simulink model "s12_euler_ssprk3_muscl_minmod_pp_ref"  (R2026a)
settings: Solver=FixedStepDiscrete  StopTime=0  FixedStep=1
model workspace (MAT data in the model file):
  S12_PP_CFLHardMax = 0.5
  S12_PP_PFloor = 1e-13
  S12_PP_RhoFloor = 1e-13
  S12_RK3_CFL = Simulink.Parameter
  S12_RK3_CFL.Value = 0.45
  S12_RK3_CFL.Complexity = 'real'
  S12_RK3_CFL.Dimensions = [1 1]
  S12_RK3_CFL.Description = 'CFL stability factor.'
  S12_RK3_CFL.DataType = 'auto'
  S12_RK3_Dx = Simulink.Parameter
  S12_RK3_Dx.Value = 0.005
  S12_RK3_Dx.Complexity = 'real'
  S12_RK3_Dx.Dimensions = [1 1]
  S12_RK3_Dx.Description = 'Uniform cell width.'
  S12_RK3_Dx.DataType = 'auto'
  S12_RK3_EndTime = Simulink.Parameter
  S12_RK3_EndTime.Value = 0.2
  S12_RK3_EndTime.Complexity = 'real'
  S12_RK3_EndTime.Dimensions = [1 1]
  S12_RK3_EndTime.Description = 'Integration end time.'
  S12_RK3_EndTime.DataType = 'auto'
  S12_RK3_Gamma = Simulink.Parameter
  S12_RK3_Gamma.Value = 1.4
  S12_RK3_Gamma.Complexity = 'real'
  S12_RK3_Gamma.Dimensions = [1 1]
  S12_RK3_Gamma.Description = 'Ratio of specific heats.'
  S12_RK3_Gamma.DataType = 'auto'
  S12_RK3_MaxSteps = Simulink.Parameter
  S12_RK3_MaxSteps.Value = 10000
  S12_RK3_MaxSteps.Complexity = 'real'
  S12_RK3_MaxSteps.Dimensions = [1 1]
  S12_RK3_MaxSteps.Description = 'Maximum accepted SSP-RK3 steps.'
  S12_RK3_MaxSteps.DataType = 'auto'
  S12_RK3_State = Simulink.Parameter
  S12_RK3_State.Value = [1 0 2.5 1 0 2.5 1 0 2.5 1 0 2.5 ... (600 elements, 3x200)]
  S12_RK3_State.Complexity = 'real'
  S12_RK3_State.Dimensions = [3 200]
  S12_RK3_State.Description = 'Classic Sod conservative state [rho; rho*u; rho*E], 3x200.'
  S12_RK3_State.DataType = 'auto'
settings Model: Creator=Jovi  LastModifiedBy=Jovi

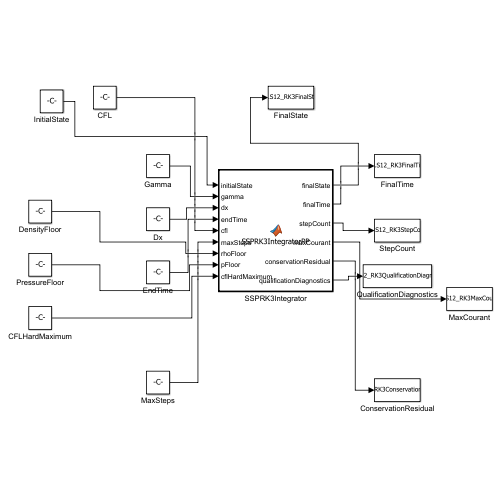
[thumbnail: Simulink's stored preview of the top-level diagram]
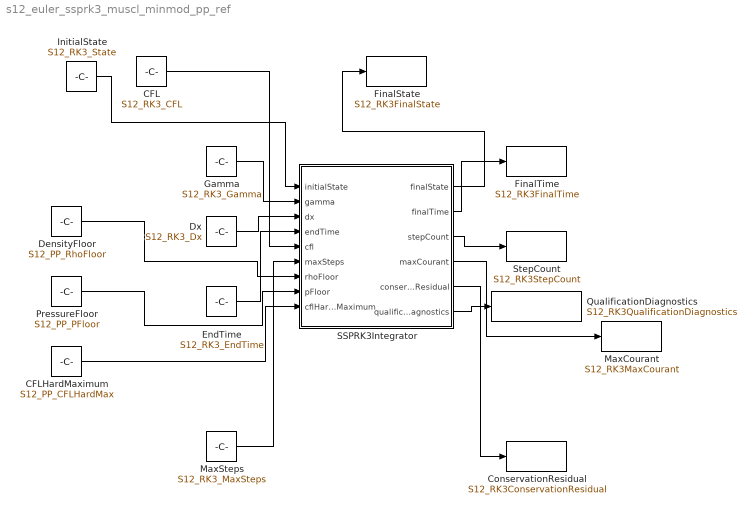
== system s12_euler_ssprk3_muscl_minmod_pp_ref ==
  CFL : Constant  Value=S12_RK3_CFL
  CFLHardMaximum : Constant  Value=S12_PP_CFLHardMax
  ConservationResidual : ToWorkspace  VariableName=S12_RK3ConservationResidual  SampleTime=-1
  DensityFloor : Constant  Value=S12_PP_RhoFloor
  Dx : Constant  Value=S12_RK3_Dx
  EndTime : Constant  Value=S12_RK3_EndTime
  FinalState : ToWorkspace  VariableName=S12_RK3FinalState  SampleTime=-1
  FinalTime : ToWorkspace  VariableName=S12_RK3FinalTime  SampleTime=-1
  Gamma : Constant  Value=S12_RK3_Gamma
  InitialState : Constant  Value=S12_RK3_State
  MaxCourant : ToWorkspace  VariableName=S12_RK3MaxCourant  SampleTime=-1
  MaxSteps : Constant  Value=S12_RK3_MaxSteps
  PressureFloor : Constant  Value=S12_PP_PFloor
  QualificationDiagnostics : ToWorkspace  VariableName=S12_RK3QualificationDiagnostics
  SSPRK3Integrator : MATLAB Function  TreatAsAtomicUnit=on
  StepCount : ToWorkspace  VariableName=S12_RK3StepCount  SampleTime=-1
  wires:
  InitialState/1 -> SSPRK3Integrator/1(initialState)
  Gamma/1 -> SSPRK3Integrator/2(gamma)
  Dx/1 -> SSPRK3Integrator/3(dx)
  EndTime/1 -> SSPRK3Integrator/4(endTime)
  CFL/1 -> SSPRK3Integrator/5(cfl)
  MaxSteps/1 -> SSPRK3Integrator/6(maxSteps)
  SSPRK3Integrator/1(finalState) -> FinalState/1
  SSPRK3Integrator/2(finalTime) -> FinalTime/1
  SSPRK3Integrator/3(stepCount) -> StepCount/1
  SSPRK3Integrator/4(maxCourant) -> MaxCourant/1
  SSPRK3Integrator/5(conservationResidual) -> ConservationResidual/1
  SSPRK3Integrator/6(qualificationDiagnostics) -> QualificationDiagnostics/1
  DensityFloor/1 -> SSPRK3Integrator/7(rhoFloor)
  PressureFloor/1 -> SSPRK3Integrator/8(pFloor)
  CFLHardMaximum/1 -> SSPRK3Integrator/9(cflHardMaximum)

== matlab function s12_euler_ssprk3_muscl_minmod_pp_ref/SSPRK3Integrator ==
  data: initialState input; finalState output; gamma input; dx input; endTime input; cfl input; maxSteps input; finalTime output; stepCount output; maxCourant output; conservationResidual output; qualificationDiagnostics output; rhoFloor input; pFloor input; cflHardMaximum input
function [finalState,finalTime,stepCount,maxCourant,conservationResidual,qualificationDiagnostics] = SSPRK3IntegratorPP(initialState,gamma,dx,endTime,cfl,maxSteps,rhoFloor,pFloor,cflHardMaximum)
%#codegen
cflTarget = 0.45;
maximumRetries = 8;
validateState(initialState,gamma,rhoFloor,pFloor);
U = initialState;
time = 0;
stepCount = 0;
maxCourant = 0;
boundaryIntegral = zeros(3,1);
qualificationDiagnostics = [inf,inf,0,0,0,0,0,0,0,0,0,1,0,0,0,1,inf,inf,inf,inf,0,0,0,0,0,inf(1,24)];
while time < endTime
    if stepCount >= maxSteps
        error('S12:Positivity:MaxSteps','PP SSP-RK3 exhausted maxSteps.');
    end
    alphaBase = stageAlpha(U,gamma);
    nominalDt = cfl*dx/alphaBase;
    dt = min(nominalDt,endTime-time);
    endClipped = dt < nominalDt;
    accepted = false;
    for attempt = 0:maximumRetries
        alpha0 = stageAlpha(U,gamma);
        if dt*alpha0/dx > cflHardMaximum
            qualificationDiagnostics(24) = qualificationDiagnostics(24)+1;
            qualificationDiagnostics(25) = qualificationDiagnostics(25)+1;
            dt = cflTarget*dx/alpha0;
            continue
        end
        [euler0,left0,right0,d0] = forwardEuler(U,gamma,dx,dt,rhoFloor,pFloor);
        U1 = euler0;
        validateState(U1,gamma,rhoFloor,pFloor);
        alpha1 = stageAlpha(U1,gamma);
        if dt*alpha1/dx > cflHardMaximum
            qualificationDiagnostics(24) = qualificationDiagnostics(24)+1;
            qualificationDiagnostics(25) = qualificationDiagnostics(25)+1;
            dt = cflTarget*dx/alpha1;
            continue
        end
        [euler1,left1,right1,d1] = forwardEuler(U1,gamma,dx,dt,rhoFloor,pFloor);
        U2 = 0.75*U+0.25*euler1;
        validateState(U2,gamma,rhoFloor,pFloor);
        alpha2 = stageAlpha(U2,gamma);
        if dt*alpha2/dx > cflHardMaximum
            qualificationDiagnostics(24) = qualificationDiagnostics(24)+1;
            qualificationDiagnostics(25) = qualificationDiagnostics(25)+1;
            dt = cflTarget*dx/alpha2;
            continue
        end
        [euler2,left2,right2,d2] = forwardEuler(U2,gamma,dx,dt,rhoFloor,pFloor);
        U3 = (1/3)*U+(2/3)*euler2;
        validateState(U3,gamma,rhoFloor,pFloor);
        qualificationDiagnostics = accumulateDiagnostics(qualificationDiagnostics,d0,d1,d2,U1,U2,U3,gamma);
        U = U3;
        boundaryIntegral = boundaryIntegral+dt*((right0-left0)/6+(right1-left1)/6+2*(right2-left2)/3);
        maxCourant = max(maxCourant,max([dt*alpha0/dx,dt*alpha1/dx,dt*alpha2/dx]));
        accepted = true;
        break
    end
    if ~accepted
        error('S12:Positivity:RetryLimit','PP SSP-RK3 exceeded the retry limit.');
    end
    qualificationDiagnostics(8) = qualificationDiagnostics(8)+double(endClipped);
    time = time+dt;
    stepCount = stepCount+1;
end
if time ~= endTime
    error('S12:Positivity:EndTime','PP SSP-RK3 did not terminate exactly.');
end
finalState = U;
finalTime = time;
conservationResidual = (dx*sum(finalState-initialState,2)+boundaryIntegral).';
end

function [stateNext,leftFlux,rightFlux,diagnostics] = forwardEuler(state,gamma,dx,dt,rhoFloor,pFloor)
cellCount = size(state,2);
alphaStage = stageAlpha(state,gamma);
lambda = dt/dx;
[rho,velocity,pressure] = recoverPrimitives(state,gamma);
slopeRho = minmodSlopes(rho);
slopeVelocity = minmodSlopes(velocity);
slopePressure = minmodSlopes(pressure);
leftPrimitive = zeros(3,cellCount);
rightPrimitive = zeros(3,cellCount);
minmodActivationCount = 0; minmodLimitedCellCount = 0;
reconstructionPPActivationCount = 0; reconstructionPPLimitedCellCount = 0;
reconstructionPPMinTheta = 1; minimumReconstructedDensity = inf; minimumReconstructedPressure = inf;
for cellIndex = 1:cellCount
    slopes = [slopeRho(cellIndex);slopeVelocity(cellIndex);slopePressure(cellIndex)];
    if cellIndex > 1 && cellIndex < cellCount
        centered = 0.5*[rho(cellIndex+1)-rho(cellIndex-1);velocity(cellIndex+1)-velocity(cellIndex-1);pressure(cellIndex+1)-pressure(cellIndex-1)];
        limited = abs(slopes-centered) > 32*eps(max([1;abs(slopes);abs(centered)]));
        minmodActivationCount = minmodActivationCount+sum(limited);
        minmodLimitedCellCount = minmodLimitedCellCount+double(any(limited));
    end
    reconstruction = s12_pp_reconstruct_primitive([rho(cellIndex);velocity(cellIndex);pressure(cellIndex)],slopes,rhoFloor,pFloor);
    leftPrimitive(:,cellIndex) = reconstruction.left;
    rightPrimitive(:,cellIndex) = reconstruction.right;
    reconstructionPPMinTheta = min(reconstructionPPMinTheta,reconstruction.theta);
    active = reconstruction.theta < 1-32*eps;
    reconstructionPPActivationCount = reconstructionPPActivationCount+double(active);
    reconstructionPPLimitedCellCount = reconstructionPPLimitedCellCount+double(active);
    minimumReconstructedDensity = min(minimumReconstructedDensity,min(reconstruction.left(1),reconstruction.right(1)));
    minimumReconstructedPressure = min(minimumReconstructedPressure,min(reconstruction.left(3),reconstruction.right(3)));
end
interfaceFlux = zeros(3,cellCount+1);
fluxPPActivationCount = 0; fluxPPLimitedInterfaceCount = 0; fluxPPMinTheta = 1;
minimumAnchorDensity = inf; minimumAnchorPressure = inf;
minimumFinalPartialDensity = inf; minimumFinalPartialPressure = inf; maximumFluxCorrectionNorm = 0;
for interfaceIndex = 1:(cellCount+1)
    if interfaceIndex == 1
        leftIndex = 1; rightIndex = 1; leftState = state(:,1); rightState = state(:,1);
    elseif interfaceIndex == cellCount+1
        leftIndex = cellCount; rightIndex = cellCount; leftState = state(:,cellCount); rightState = state(:,cellCount);
    else
        leftIndex = interfaceIndex-1; rightIndex = interfaceIndex;
        leftState = conservativeFromPrimitives(rightPrimitive(1,leftIndex),rightPrimitive(2,leftIndex),rightPrimitive(3,leftIndex),gamma);
        rightState = conservativeFromPrimitives(leftPrimitive(1,rightIndex),leftPrimitive(2,rightIndex),leftPrimitive(3,rightIndex),gamma);
    end
    highFlux = hllcFlux(leftState,rightState,gamma);
    lowFlux = s12_pp_global_lf_flux(state(:,leftIndex),state(:,rightIndex),gamma,alphaStage);
    limitedFlux = s12_pp_limit_interface_flux(state(:,leftIndex),state(:,rightIndex),highFlux,lowFlux,lambda,gamma,rhoFloor,pFloor);
    interfaceFlux(:,interfaceIndex) = limitedFlux.flux;
    fluxPPMinTheta = min(fluxPPMinTheta,limitedFlux.theta);
    active = limitedFlux.theta < 1-32*eps;
    fluxPPActivationCount = fluxPPActivationCount+double(active);
    fluxPPLimitedInterfaceCount = fluxPPLimitedInterfaceCount+double(active);
    minimumAnchorDensity = min(minimumAnchorDensity,min(limitedFlux.low_left_partial(1),limitedFlux.low_right_partial(1)));
    minimumAnchorPressure = min(minimumAnchorPressure,min(pressureOf(limitedFlux.low_left_partial,gamma),pressureOf(limitedFlux.low_right_partial,gamma)));
    minimumFinalPartialDensity = min(minimumFinalPartialDensity,min(limitedFlux.left_partial(1),limitedFlux.right_partial(1)));
    minimumFinalPartialPressure = min(minimumFinalPartialPressure,min(pressureOf(limitedFlux.left_partial,gamma),pressureOf(limitedFlux.right_partial,gamma)));
    maximumFluxCorrectionNorm = max(maximumFluxCorrectionNorm,limitedFlux.correction_norm);
end
stateNext = zeros(size(state));
for cellIndex = 1:cellCount
    stateNext(:,cellIndex) = state(:,cellIndex)-lambda*(interfaceFlux(:,cellIndex+1)-interfaceFlux(:,cellIndex));
end
validateState(stateNext,gamma,rhoFloor,pFloor);
leftFlux = interfaceFlux(:,1); rightFlux = interfaceFlux(:,end);
diagnostics = [minmodActivationCount,minmodLimitedCellCount,max(cellCount-2,0),reconstructionPPActivationCount,reconstructionPPLimitedCellCount,reconstructionPPMinTheta,minimumReconstructedDensity,minimumReconstructedPressure,0,fluxPPActivationCount,fluxPPLimitedInterfaceCount,cellCount+1,fluxPPMinTheta,minimumAnchorDensity,minimumAnchorPressure,minimumFinalPartialDensity,minimumFinalPartialPressure,alphaStage,maximumFluxCorrectionNorm,0];
end

function total = accumulateDiagnostics(total,d0,d1,d2,U1,U2,U3,gamma)
for diagnostics = [d0(:),d1(:),d2(:)]
    total(1)=min(total(1),diagnostics(7)); total(2)=min(total(2),diagnostics(8)); total(3)=total(3)+diagnostics(9);
    total(4)=total(4)+diagnostics(1); total(5)=total(5)+diagnostics(2); total(6)=total(6)+diagnostics(3); total(7)=total(7)+1;
    total(9)=total(9)+diagnostics(4); total(10)=total(10)+diagnostics(5); total(11)=total(11)+diagnostics(3); total(12)=min(total(12),diagnostics(6));
    total(13)=total(13)+diagnostics(10); total(14)=total(14)+diagnostics(11); total(15)=total(15)+diagnostics(12); total(16)=min(total(16),diagnostics(13));
    total(17)=min(total(17),diagnostics(14)); total(18)=min(total(18),diagnostics(15)); total(19)=min(total(19),diagnostics(16)); total(20)=min(total(20),diagnostics(17));
    total(21)=max(total(21),diagnostics(18)); total(22)=max(total(22),diagnostics(19)); total(23)=total(23)+diagnostics(20);
end
[rho1,~,p1]=recoverPrimitives(U1,gamma); [rho2,~,p2]=recoverPrimitives(U2,gamma); [rho3,~,p3]=recoverPrimitives(U3,gamma);
total(26)=min(total(26),min(rho1)); total(27)=min(total(27),min(p1)); total(28)=min(total(28),min(rho2)); total(29)=min(total(29),min(p2)); total(30)=min(total(30),min(rho3)); total(31)=min(total(31),min(p3));
stageDiagnostics=[d0(:),d1(:),d2(:)];
for stageIndex=1:3
    total(31+stageIndex)=min(total(31+stageIndex),stageDiagnostics(7,stageIndex));
    total(34+stageIndex)=min(total(34+stageIndex),stageDiagnostics(8,stageIndex));
    total(37+stageIndex)=min(total(37+stageIndex),stageDiagnostics(14,stageIndex));
    total(40+stageIndex)=min(total(40+stageIndex),stageDiagnostics(15,stageIndex));
    total(43+stageIndex)=min(total(43+stageIndex),stageDiagnostics(16,stageIndex));
    total(46+stageIndex)=min(total(46+stageIndex),stageDiagnostics(17,stageIndex));
end
end

function alpha = stageAlpha(state,gamma)
[rho,velocity,pressure]=recoverPrimitives(state,gamma); alpha=max(abs(velocity)+sqrt(gamma*pressure./rho));
end
function validateState(state,gamma,rhoFloor,pFloor)
[rho,~,pressure]=recoverPrimitives(state,gamma); if any(~isfinite(state(:))) || any(rho<rhoFloor) || any(pressure<pFloor), error('S12:Positivity:InvalidStage','A PP stage violated the configured floors.'); end
end
function [rho,velocity,pressure]=recoverPrimitives(state,gamma)
rho=state(1,:); velocity=state(2,:)./rho; pressure=(gamma-1)*(state(3,:)-0.5*rho.*velocity.^2);
end
function value=pressureOf(state,gamma)
rho=state(1); velocity=state(2)/rho; value=(gamma-1)*(state(3)-0.5*rho*velocity^2);
end
function state=conservativeFromPrimitives(rho,velocity,pressure,gamma)
state=[rho;rho*velocity;pressure/(gamma-1)+0.5*rho*velocity^2];
end
function slopes=minmodSlopes(values)
cellCount=numel(values); slopes=zeros(size(values)); for cellIndex=2:(cellCount-1), slopes(cellIndex)=minmod(values(cellIndex)-values(cellIndex-1),values(cellIndex+1)-values(cellIndex)); end
end
function value=minmod(leftDelta,rightDelta)
if leftDelta*rightDelta<=0, value=0; elseif abs(leftDelta)<=abs(rightDelta), value=leftDelta; else, value=rightDelta; end
end
function flux=hllcFlux(stateL,stateR,gamma)
rhoL=stateL(1);rhoR=stateR(1);uL=stateL(2)/rhoL;uR=stateR(2)/rhoR;energyL=stateL(3);energyR=stateR(3);pL=(gamma-1)*(energyL-0.5*rhoL*uL*uL);pR=(gamma-1)*(energyR-0.5*rhoR*uR*uR);soundL=sqrt(gamma*pL/rhoL);soundR=sqrt(gamma*pR/rhoR);sL=min(uL-soundL,uR-soundR);sR=max(uL+soundL,uR+soundR);sM=(pR-pL+rhoL*uL*(sL-uL)-rhoR*uR*(sR-uR))/(rhoL*(sL-uL)-rhoR*(sR-uR));fluxL=[rhoL*uL;rhoL*uL*uL+pL;uL*(energyL+pL)];fluxR=[rhoR*uR;rhoR*uR*uR+pR;uR*(energyR+pR)];
if sL>=0, flux=fluxL; elseif sM>=0, rhoStarL=rhoL*(sL-uL)/(sL-sM);energyStarL=rhoStarL*(energyL/rhoL+(sM-uL)*(sM+pL/(rhoL*(sL-uL))));flux=fluxL+sL*([rhoStarL;rhoStarL*sM;energyStarL]-stateL); elseif sR>0, rhoStarR=rhoR*(sR-uR)/(sR-sM);energyStarR=rhoStarR*(energyR/rhoR+(sM-uR)*(sM+pR/(rhoR*(sR-uR))));flux=fluxR+sR*([rhoStarR;rhoStarR*sM;energyStarR]-stateR); else, flux=fluxR; end
end
